simulink model "Boat_sim"  (Simulink 7.5)
settings: Solver=FixedStepDiscrete  StartTime=0.0  StopTime=1000  FixedStep=.01  RelTol=1e-3
InitFcn:
  | boat_constants
values from neighbouring files (symbols this model uses):
  C_d_sea_surge = 340    [boat_constants.m]
  d_prop = .4572    (= 0.4572)    [boat_constants.m]
  figure8_waypoints = int32([ ... (first row only)    [boat_constants.m]
  InitialPoint = 0    [boat_constants.m]    (also in l2plus.m)
  IPStar = 0    [boat_constants.m]    (also in l2plus.m)
  ISA_g = 9.815    [boat_constants.m]
  K_t = 0.5    [boat_constants.m]
  mass = 550    [boat_constants.m]
  MaxDwnPthStar = 1    [boat_constants.m]    (also in l2plus.m)
  OC2max = 49999    [boat_constants.m]    (also in simulation_constants.m)
  phi_0 = 0    [boat_constants.m]    (also in simulation_constants.m)
  rho_w = 1.03e3    (= 1030)    [boat_constants.m]
  sampling_waypoints = int32([ ... (first row only)    [boat_constants.m]
  switchDistance = 4    [boat_constants.m]    (also in l2plus.m)
  T_step = 0.01    [boat_constants.m]    (also in common.m)
  tanIntercept = tan( 45*pi/180 )    [boat_constants.m]    (also in l2plus.m)
  test_waypoints = int32([ ... (first row only)    [boat_constants.m]
  TStar = single(4.5)    [boat_constants.m]    (also in l2plus.m = single(2))
  Turn2Track = 0    [boat_constants.m]    (also in l2plus.m)
  wheelbase = 3.27    [boat_constants.m]
undefined symbols (not defined in the file or in its folder): clock, DiscIntNeverNeededParam, Earth, serial, WGS84
libraries: simulink x25, uSimLib x4, instrumentlib x3, aerolibconvert2 x2, aerolibtransform2 x1, aerolibanimutils x1, simulink_need_slupdate x1
(part 2 of 3)

== system Boat_sim/Subsystem/Log state data to workspace ==
  L2 : Inport
  gPos : Inport  Port=2
  head : Inport  Port=3
  lPos : Inport  Port=4
  vel : Inport  Port=5
  Build HIL sentence : Subsystem
  Pack : Stateflow chart  TreatAsAtomicUnit=on
  To Workspace2 : ToWorkspace  VariableName=state  SampleTime=-1  SaveFormat=Array
  wires:
  Pack/1(y) -> Build HIL sentence/1(data)
  Build HIL sentence/1(sent) -> To Workspace2/1
  L2/1 -> Pack/1(L2)
  gPos/1 -> Pack/2(gPos)
  head/1 -> Pack/3(head)
  lPos/1 -> Pack/4(lPos)
  vel/1 -> Pack/5(vel)

== system Boat_sim/Subsystem/Map from to 655..347 to -.7854..+.7854 ==
  In1 : Inport
  Bias1 : Bias  Bias=-501
  Data Type Conversion : DataTypeConversion  OutDataTypeMode=single  OutDataType=fixdt(1, 16)  OutScaling=2^0  OutDataTypeStr=single
  Gain : Gain  Gain=1/196  ParameterDataType=fixdt(1, 16)  ParameterScaling=2^0  OutDataType=fixdt(1, 16)  OutScaling=2^0
  Out1 : Outport
  wires:
  In1/1 -> Data Type Conversion/1
  Gain/1 -> Out1/1
  Bias1/1 -> Gain/1
  Data Type Conversion/1 -> Bias1/1

== system Boat_sim/Plant/Actuator Dynamics/Enabled Subsystem ==
  note: Map from 0,1 to -.02,.02
  In1 : Inport  OutDataType=fixdt(1, 16)  OutScaling=2^0
  Enable : EnablePort
  Bias : Bias  Bias=-1
  Data Type Conversion3 : DataTypeConversion  OutDataTypeMode=single  OutDataType=sfix(16)  OutScaling=2^0  OutDataTypeStr=single
  Gain : Gain  Gain=2  ParameterDataType=fixdt(1, 16)  ParameterScaling=2^0  OutDataTypeMode=double  OutDataType=fixdt(1, 16)  OutScaling=2^0  OutDataTypeStr=double
  Gain1 : Gain  Gain=.05  ParameterDataType=fixdt(1, 16)  ParameterScaling=2^0  OutDataType=fixdt(1, 16)  OutScaling=2^0
  Out1 : Outport  OutDataType=fixdt(1, 16)  OutScaling=2^0
  wires:
  In1/1 -> Data Type Conversion3/1
  Gain/1 -> Bias/1
  Bias/1 -> Gain1/1
  Gain1/1 -> Out1/1
  Data Type Conversion3/1 -> Gain/1

== system Boat_sim/Plant/Actuator Dynamics/Enabled Subsystem1 ==
  note: Map from 0,1 to -.5,.5
  In1 : Inport  OutDataType=fixdt(1, 16)  OutScaling=2^0
  Bias : Bias  Bias=-1
  Data Type Conversion : DataTypeConversion  OutDataTypeMode=single  OutDataType=fixdt(1, 16)  OutScaling=2^0  OutDataTypeStr=single
  Gain : Gain  Gain=2  ParameterDataType=fixdt(1, 16)  ParameterScaling=2^0  OutDataTypeMode=double  OutDataType=fixdt(1, 16)  OutScaling=2^0  OutDataTypeStr=double
  Shift Arithmetic : simulink/Logic and Bit Operations/Shift Arithmetic  SystemSampleTime=-1  nBitShiftRight=1  nBinPtShiftRight=0
  Out1 : Outport  OutDataType=fixdt(1, 16)  OutScaling=2^0
  wires:
  In1/1 -> Data Type Conversion/1
  Gain/1 -> Bias/1
  Bias/1 -> Shift Arithmetic/1
  Shift Arithmetic/1 -> Out1/1
  Data Type Conversion/1 -> Gain/1

== system Boat_sim/Plant/Actuator Dynamics/Second Order Linear Actuator1 ==
  Ac_dem : Inport  OutDataType=sfix(16)  OutScaling=2^0
  2*zeta * wn : Gain  Gain=2.0 * z_fin* wn_fin  ParameterDataType=sfix(16)  ParameterScaling=2^0  OutDataType=sfix(16)  OutScaling=2^0  SaturateOnIntegerOverflow=on  OutDataTypeStr=Inherit: Same as input  ParamDataTypeStr=Inherit: Same as input
  Discrete-Time Integrator1 : DiscreteIntegrator  SampleTime=-1  OutDataType=fixdt(1, 16)  OutScaling=2^0  UpperSaturationLimit=1  LowerSaturationLimit=-1  ICPrevOutput=DiscIntNeverNeededParam  ICPrevScaledInput=DiscIntNeverNeededParam
  Discrete-Time Integrator2 : DiscreteIntegrator  SampleTime=-1  OutDataType=fixdt(1, 16)  OutScaling=2^0  UpperSaturationLimit=1  LowerSaturationLimit=-1  ICPrevOutput=DiscIntNeverNeededParam  ICPrevScaledInput=DiscIntNeverNeededParam
  Sum2 : Sum  Inputs=|+-  OutDataType=sfix(16)  OutScaling=2^0  SaturateOnIntegerOverflow=on  InputSameDT=on  OutDataTypeStr=Inherit: Same as first input
  Sum3 : Sum  Inputs=|+-  OutDataType=sfix(16)  OutScaling=2^0  SaturateOnIntegerOverflow=on  InputSameDT=on  OutDataTypeStr=Inherit: Same as first input
  wn^2 : Gain  Gain=wn_fin* wn_fin  ParameterDataType=sfix(16)  ParameterScaling=2^0  OutDataType=sfix(16)  OutScaling=2^0  SaturateOnIntegerOverflow=on  OutDataTypeStr=Inherit: Same as input  ParamDataTypeStr=Inherit: Same as input
  Ac_ac : Outport  OutDataType=sfix(16)  OutScaling=2^0  InitialOutput=0
  wires:
  Discrete-Time Integrator1/1 -> Ac_ac/1, Sum3/2
  wn^2/1 -> Sum2/1
  Sum2/1 -> Discrete-Time Integrator2/1
  Discrete-Time Integrator2/1 -> 2*zeta * wn/1, Discrete-Time Integrator1/1
  2*zeta * wn/1 -> Sum2/2
  Ac_dem/1 -> Sum3/1
  Sum3/1 -> wn^2/1

== system Boat_sim/Plant/Actuator Dynamics/Second Order Linear Actuator2 ==
  Ac_dem : Inport  OutDataType=sfix(16)  OutScaling=2^0
  2*zeta * wn : Gain  Gain=2.0 * z_fin* wn_fin  ParameterDataType=sfix(16)  ParameterScaling=2^0  OutDataType=sfix(16)  OutScaling=2^0  SaturateOnIntegerOverflow=on  OutDataTypeStr=Inherit: Same as input  ParamDataTypeStr=Inherit: Same as input
  Discrete-Time Integrator1 : DiscreteIntegrator  SampleTime=-1  OutDataType=fixdt(1, 16)  OutScaling=2^0  UpperSaturationLimit=1  LowerSaturationLimit=-1  ICPrevOutput=DiscIntNeverNeededParam  ICPrevScaledInput=DiscIntNeverNeededParam
  Discrete-Time Integrator2 : DiscreteIntegrator  SampleTime=-1  OutDataType=fixdt(1, 16)  OutScaling=2^0  UpperSaturationLimit=1  LowerSaturationLimit=-1  ICPrevOutput=DiscIntNeverNeededParam  ICPrevScaledInput=DiscIntNeverNeededParam
  Sum2 : Sum  Inputs=|+-  OutDataType=sfix(16)  OutScaling=2^0  SaturateOnIntegerOverflow=on  InputSameDT=on  OutDataTypeStr=Inherit: Same as first input
  Sum3 : Sum  Inputs=|+-  OutDataType=sfix(16)  OutScaling=2^0  SaturateOnIntegerOverflow=on  InputSameDT=on  OutDataTypeStr=Inherit: Same as first input
  wn^2 : Gain  Gain=wn_fin* wn_fin  ParameterDataType=sfix(16)  ParameterScaling=2^0  OutDataType=sfix(16)  OutScaling=2^0  SaturateOnIntegerOverflow=on  OutDataTypeStr=Inherit: Same as input  ParamDataTypeStr=Inherit: Same as input
  Ac_ac : Outport  OutDataType=sfix(16)  OutScaling=2^0  InitialOutput=0
  wires:
  Discrete-Time Integrator1/1 -> Ac_ac/1, Sum3/2
  wn^2/1 -> Sum2/1
  Sum2/1 -> Discrete-Time Integrator2/1
  Discrete-Time Integrator2/1 -> 2*zeta * wn/1, Discrete-Time Integrator1/1
  2*zeta * wn/1 -> Sum2/2
  Ac_dem/1 -> Sum3/1
  Sum3/1 -> wn^2/1

== system Boat_sim/Plant/Actuator Dynamics/Second Order Linear Actuator3 ==
  Ac_dem : Inport  OutDataType=sfix(16)  OutScaling=2^0
  2*zeta * wn : Gain  Gain=2.0 * z_fin* wn_fin  ParameterDataType=sfix(16)  ParameterScaling=2^0  OutDataType=sfix(16)  OutScaling=2^0  SaturateOnIntegerOverflow=on  OutDataTypeStr=Inherit: Same as input  ParamDataTypeStr=Inherit: Same as input
  Discrete-Time Integrator1 : DiscreteIntegrator  SampleTime=-1  OutDataType=fixdt(1, 16)  OutScaling=2^0  UpperSaturationLimit=1  LowerSaturationLimit=-1  ICPrevOutput=DiscIntNeverNeededParam  ICPrevScaledInput=DiscIntNeverNeededParam
  Discrete-Time Integrator2 : DiscreteIntegrator  SampleTime=-1  OutDataType=fixdt(1, 16)  OutScaling=2^0  UpperSaturationLimit=1  LowerSaturationLimit=-1  ICPrevOutput=DiscIntNeverNeededParam  ICPrevScaledInput=DiscIntNeverNeededParam
  Sum2 : Sum  Inputs=|+-  OutDataType=sfix(16)  OutScaling=2^0  SaturateOnIntegerOverflow=on  InputSameDT=on  OutDataTypeStr=Inherit: Same as first input
  Sum3 : Sum  Inputs=|+-  OutDataType=sfix(16)  OutScaling=2^0  SaturateOnIntegerOverflow=on  InputSameDT=on  OutDataTypeStr=Inherit: Same as first input
  wn^2 : Gain  Gain=wn_fin* wn_fin  ParameterDataType=sfix(16)  ParameterScaling=2^0  OutDataType=sfix(16)  OutScaling=2^0  SaturateOnIntegerOverflow=on  OutDataTypeStr=Inherit: Same as input  ParamDataTypeStr=Inherit: Same as input
  Ac_ac : Outport  OutDataType=sfix(16)  OutScaling=2^0  InitialOutput=0
  wires:
  Discrete-Time Integrator1/1 -> Ac_ac/1, Sum3/2
  wn^2/1 -> Sum2/1
  Sum2/1 -> Discrete-Time Integrator2/1
  Discrete-Time Integrator2/1 -> 2*zeta * wn/1, Discrete-Time Integrator1/1
  2*zeta * wn/1 -> Sum2/2
  Ac_dem/1 -> Sum3/1
  Sum3/1 -> wn^2/1

== system Boat_sim/Plant/Actuator Dynamics/Subsystem ==
  note: This block stores the throttle speed. As the speed is only set intermittently,
      | the speed is saved to memory and constrantly output. It is only updated when
      | a properly packaged CAN message is delivered based on its ID and the trigger
      | bit.
  In1 : Inport
  Bus Selector2 : BusSelector  OutputSignals=identifier,trigger,data
  Data Store Memory : DataStoreMemory  DataStoreName=throttle_speed  WriteAfterWriteMsg=warning  WriteAfterReadMsg=warning  DataType=double  OutDataType=fixdt(1, 16)  OutScaling=2^0  OutDataTypeStr=double
  Data Store Read : DataStoreRead  Priority=2  DataStoreName=throttle_speed  SampleTime=T_step
  Data Type Conversion : DataTypeConversion  OutDataTypeMode=uint32  OutDataType=fixdt(1, 16)  OutScaling=2^0  OutDataTypeStr=uint32  RndMeth=Simplest
  If : If  NumInputs=2  IfExpression=u1 == hex2dec('301')  ShowElse=off
  If Action Subsystem : Subsystem  Priority=1  TreatAsAtomicUnit=on
  Scope1 : Scope
      settings: YMin=971.85  YMax=1074.15  SaveName=ScopeData2
  To Workspace : ToWorkspace  VariableName=t_data  SampleTime=-1  SaveFormat=Structure
  Out1 : Outport
  wires:
  In1/1 -> Bus Selector2/1
  Data Store Read/1 -> Out1/1, Scope1/1
  Bus Selector2/1 -> If/1  "<identifier>"
  Bus Selector2/2 -> Data Type Conversion/1  "<trigger>"
  If/1 -> If Action Subsystem/Action
  Bus Selector2/3 -> If Action Subsystem/1(In1), To Workspace/1  "<data>"
  Data Type Conversion/1 -> If/2

== system Boat_sim/Plant/Actuator Dynamics/Subsystem1 ==
  note: This block simulates the stepper motor driver board logic for stepping the motor.
      | The enable line must be low, it's active low, and a pulse train must be received. As
      | the enable line is always low to provide holding torque, the lines specifying a pulse
      | train must are therefore checked to confirm that the rudder should be moving. The
      | exact values of both the up and period signals are unimportant, so they're just
      | compared to zero.
  e : Inport
  u : Inport  Port=2
  p : Inport  Port=3
  Compare To Zero : simulink/Logic and Bit Operations/Compare To Zero  SystemSampleTime=-1  relop=~=  LogicOutDataTypeMode=boolean
  Compare To Zero1 : simulink/Logic and Bit Operations/Compare To Zero  SystemSampleTime=-1  relop=~=  LogicOutDataTypeMode=boolean
  Logical Operator : Logic  Operator=NOT  AllPortsSameDT=off  OutDataTypeMode=boolean  LogicDataType=fixdt(0, 8)  OutDataTypeStr=boolean
  Logical Operator1 : Logic  Inputs=3  AllPortsSameDT=off  OutDataTypeMode=boolean  LogicDataType=fixdt(0, 8)  OutDataTypeStr=boolean
  Out1 : Outport
  wires:
  e/1 -> Logical Operator/1
  Logical Operator1/1 -> Out1/1
  p/1 -> Compare To Zero/1
  Compare To Zero/1 -> Logical Operator1/3
  Compare To Zero1/1 -> Logical Operator1/2
  u/1 -> Compare To Zero1/1
  Logical Operator/1 -> Logical Operator1/1

== system Boat_sim/Plant/Generate sensor data from actuator position/Map from +-.7854 to 655..347 ==
  In1 : Inport
  Bias1 : Bias  Bias=501
  Data Type Conversion : DataTypeConversion  OutDataTypeMode=uint16  OutDataType=fixdt(1, 16)  OutScaling=2^0  OutDataTypeStr=uint16
  Gain1 : Gain  Gain=196  ParameterDataType=fixdt(1, 16)  ParameterScaling=2^0  OutDataType=fixdt(1, 16)  OutScaling=2^0
  Out1 : Outport
  wires:
  Bias1/1 -> Data Type Conversion/1
  In1/1 -> Gain1/1
  Data Type Conversion/1 -> Out1/1
  Gain1/1 -> Bias1/1

== system Boat_sim/Plant/Generate sensor data from actuator position/Map from -1..1 to -1023..1023 ==
  In1 : Inport
  Data Type Conversion : DataTypeConversion  OutDataTypeMode=int16  OutDataType=fixdt(1, 16)  OutScaling=2^0  OutDataTypeStr=int16  RndMeth=Simplest
  Gain : Gain  Gain=1023  ParameterDataType=fixdt(1, 16)  ParameterScaling=2^0  OutDataType=fixdt(1, 16)  OutScaling=2^0
  Out1 : Outport
  wires:
  Gain/1 -> Data Type Conversion/1
  In1/1 -> Gain/1
  Data Type Conversion/1 -> Out1/1

== system Boat_sim/Plant/Generate sensor data from actuator position/Map from -1..1 to 620..313 ==
  In1 : Inport
  Bias : Bias  Bias=466.5
  Data Type Conversion : DataTypeConversion  OutDataTypeMode=uint16  OutDataType=fixdt(1, 16)  OutScaling=2^0  OutDataTypeStr=uint16
  Gain : Gain  Gain=-153.5  ParameterDataType=fixdt(1, 16)  ParameterScaling=2^0  OutDataType=fixdt(1, 16)  OutScaling=2^0
  Out1 : Outport
  wires:
  Data Type Conversion/1 -> Out1/1
  In1/1 -> Gain/1
  Bias/1 -> Data Type Conversion/1
  Gain/1 -> Bias/1

== system Boat_sim/Subsystem/Autonomous Controller/Ballast Command ==
  Bus Creator : BusCreator  Inputs=2
  Constant : Constant  Value=0  OutDataTypeMode=boolean  OutDataType=fixdt(1, 16)  OutScaling=2^0  OutDataTypeStr=boolean
  Constant1 : Constant  Value=0  OutDataTypeMode=boolean  OutDataType=fixdt(1, 16)  OutScaling=2^0  OutDataTypeStr=boolean
  c_ballast : Outport
  wires:
  Constant1/1 -> Bus Creator/2  "direction"
  Constant/1 -> Bus Creator/1  "enable"
  Bus Creator/1 -> c_ballast/1

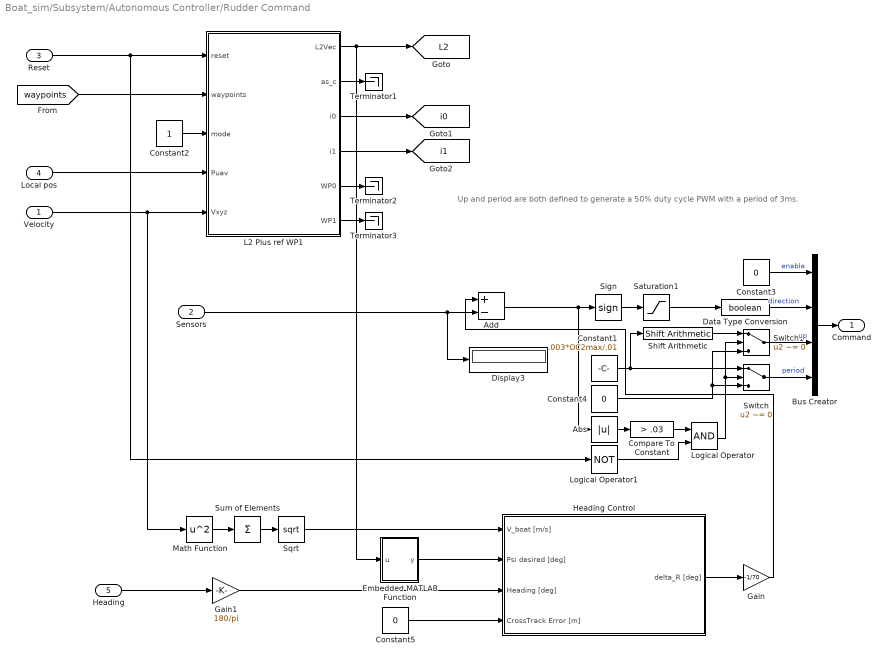
== system Boat_sim/Subsystem/Autonomous Controller/Rudder Command ==
  note: Up and period are both defined to generate a 50% duty cycle PWM with
      | a period of 3ms.
  Velocity : Inport
  Sensors : Inport  Port=2
  Reset : Inport  Port=3
  Local pos : Inport  Port=4
  Heading : Inport  Port=5
  Abs : Abs  OutDataType=fixdt(1, 16)  OutScaling=2^0
  Add : Sum  Inputs=+-  OutDataType=fixdt(1, 16)  OutScaling=2^-10
  Bus Creator : BusCreator
  Compare To Constant : simulink/Logic and Bit Operations/Compare To Constant  SystemSampleTime=-1  relop=>  const=.03  LogicOutDataTypeMode=boolean
  Constant1 : Constant  Value=.003*OC2max/.01  OutDataTypeMode=uint16  OutDataType=sfix(16)  OutScaling=2^0  OutDataTypeStr=uint16
  Constant2 : Constant  OutDataTypeMode=uint8  OutDataType=sfix(16)  OutScaling=2^0  OutDataTypeStr=uint8
  Constant3 : Constant  Value=0  OutDataTypeMode=boolean  OutDataType=sfix(16)  OutScaling=2^0  OutDataTypeStr=boolean
  Constant4 : Constant  Value=0  OutDataTypeMode=uint16  OutDataType=sfix(16)  OutScaling=2^0  OutDataTypeStr=uint16
  Constant5 : Constant  Value=0  OutDataTypeMode=uint8  OutDataType=sfix(16)  OutScaling=2^0  OutDataTypeStr=uint8
  Data Type Conversion : DataTypeConversion  OutDataTypeMode=boolean  OutDataType=fixdt(1, 16)  OutScaling=2^0  OutDataTypeStr=boolean  RndMeth=Simplest
  Display3 : Display
  Embedded MATLAB Function : Stateflow chart  TreatAsAtomicUnit=on
  Gain : Gain  Gain=-1/70  ParameterDataType=fixdt(1, 16)  ParameterScaling=2^0  OutDataType=fixdt(1, 16)  OutScaling=2^0
  Gain1 : Gain  Gain=180/pi  ParameterDataType=fixdt(1, 16)  ParameterScaling=2^0  OutDataType=fixdt(1, 16)  OutScaling=2^0
  Heading Control : Subsystem
  L2 Plus ref WP1 : Stateflow chart  TreatAsAtomicUnit=on
  Logical Operator : Logic  AllPortsSameDT=off  OutDataTypeMode=boolean  LogicDataType=fixdt(0, 8)  OutDataTypeStr=boolean
  Logical Operator1 : Logic  Operator=NOT  Inputs=1  AllPortsSameDT=off  OutDataTypeMode=boolean  LogicDataType=fixdt(0, 8)  OutDataTypeStr=boolean
  Math Function : Math  Operator=square  OutDataType=fixdt(1, 16)  OutScaling=2^0  SaturateOnIntegerOverflow=on
  Saturation1 : Saturate  UpperLimit=1  LowerLimit=0  OutDataTypeStr=Inherit: Inherit via back propagation
  Shift Arithmetic : simulink/Logic and Bit Operations/Shift Arithmetic  SystemSampleTime=-1  nBitShiftRight=1  nBinPtShiftRight=0
  Sign : Signum
  Sqrt : Sqrt  SaturateOnIntegerOverflow=on
  Sum of Elements : Sum  Inputs=+  OutDataType=fixdt(1, 16)  OutScaling=2^-10
  Switch : Switch  Criteria=u2 ~= 0  OutDataType=fixdt(1, 16)  OutScaling=2^0
  Switch1 : Switch  Criteria=u2 ~= 0  OutDataType=fixdt(1, 16)  OutScaling=2^0
  Terminator1 : Terminator
  Terminator2 : Terminator
  Terminator3 : Terminator
  Command : Outport
  tag scope: L2=global, i0=global, i1=global
  wires:
  Add/1 -> Abs/1, Sign/1
  Embedded MATLAB Function/1(y) -> Heading Control/2(Psi desired [deg])
  Gain1/1 -> Heading Control/3(Heading [deg])
  Gain/1 -> Add/1
  Heading Control/1(delta_R [deg]) -> Gain/1
  Sum of Elements/1 -> Sqrt/1
  Math Function/1 -> Sum of Elements/1
  Sqrt/1 -> Heading Control/1(V_boat [m/s])
  Constant5/1 -> Heading Control/4(CrossTrack Error [m])
  Heading/1 -> Gain1/1
  [waypoints] -> L2 Plus ref WP1/2(waypoints)
  Logical Operator1/1 -> Logical Operator/2
  Logical Operator/1 -> Switch1/2, Switch/2
  Compare To Constant/1 -> Logical Operator/1
  L2 Plus ref WP1/4(i1) -> [i1]
  L2 Plus ref WP1/3(i0) -> [i0]
  Local pos/1 -> L2 Plus ref WP1/4(Puav)
  Reset/1 -> Logical Operator1/1, L2 Plus ref WP1/1(reset)
  Constant4/1 -> Switch1/3, Switch/3
  Switch1/1 -> Bus Creator/3  "up"
  Switch/1 -> Bus Creator/4  "period"
  Shift Arithmetic/1 -> Switch1/1
  Abs/1 -> Compare To Constant/1
  Constant1/1 -> Switch/1, Shift Arithmetic/1
  Constant3/1 -> Bus Creator/1  "enable"
  Velocity/1 -> Math Function/1, L2 Plus ref WP1/5(Vxyz)
  L2 Plus ref WP1/1(L2Vec) -> Embedded MATLAB Function/1(u), [L2]
  Constant2/1 -> L2 Plus ref WP1/3(mode)
  Sign/1 -> Saturation1/1
  Saturation1/1 -> Data Type Conversion/1
  Bus Creator/1 -> Command/1
  Sensors/1 -> Add/2, Display3/1
  Data Type Conversion/1 -> Bus Creator/2  "direction"
  L2 Plus ref WP1/2(as_c) -> Terminator1/1
  L2 Plus ref WP1/5(WP0) -> Terminator2/1
  L2 Plus ref WP1/6(WP1) -> Terminator3/1

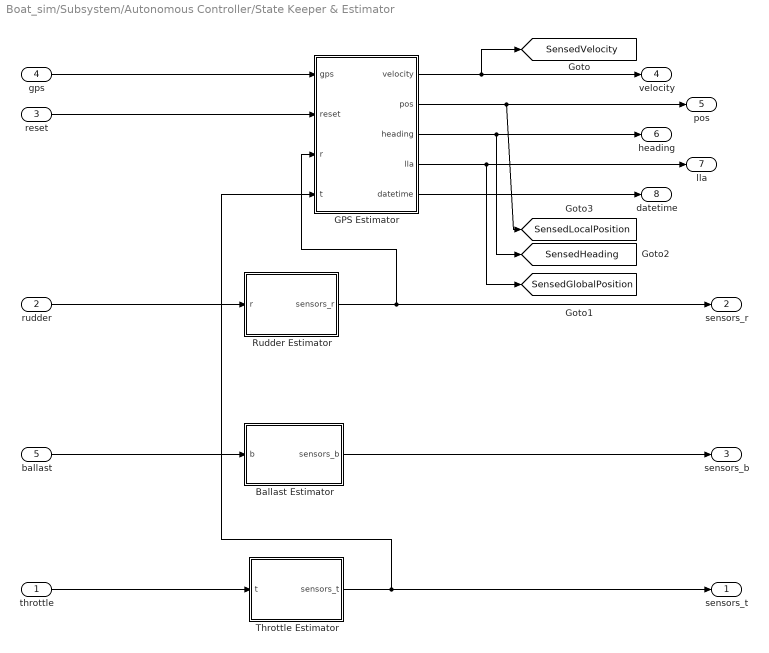
== system Boat_sim/Subsystem/Autonomous Controller/State Keeper & Estimator ==
  throttle : Inport
  rudder : Inport  Port=2
  reset : Inport  Port=3
  gps : Inport  Port=4
  ballast : Inport  Port=5
  Ballast Estimator : Subsystem
  GPS Estimator : Subsystem
  Rudder Estimator : Subsystem
  Throttle Estimator : Subsystem
  sensors_t : Outport
  sensors_r : Outport  Port=2
  sensors_b : Outport  Port=3
  velocity : Outport  Port=4
  pos : Outport  Port=5
  heading : Outport  Port=6
  lla : Outport  Port=7
  datetime : Outport  Port=8
  tag scope: SensedGlobalPosition=global, SensedHeading=global, SensedLocalPosition=global, SensedVelocity=global
  wires:
  Throttle Estimator/1(sensors_t) -> GPS Estimator/4(t), sensors_t/1
  Ballast Estimator/1(sensors_b) -> sensors_b/1
  Rudder Estimator/1(sensors_r) -> GPS Estimator/3(r), sensors_r/1
  GPS Estimator/5(datetime) -> datetime/1
  GPS Estimator/4(lla) -> lla/1, [SensedGlobalPosition]
  GPS Estimator/3(heading) -> [SensedHeading], heading/1
  GPS Estimator/2(pos) -> [SensedLocalPosition], pos/1
  gps/1 -> GPS Estimator/1(gps)
  GPS Estimator/1(velocity) -> [SensedVelocity], velocity/1
  reset/1 -> GPS Estimator/2(reset)
  throttle/1 -> Throttle Estimator/1(t)
  ballast/1 -> Ballast Estimator/1(b)
  rudder/1 -> Rudder Estimator/1(r)

== system Boat_sim/Subsystem/Autonomous Controller/Throttle Command ==
  sensors : Inport
  reset : Inport  Port=2
  Bus Creator : BusCreator
  Constant1 : Constant  Value=0  OutDataTypeMode=int16  OutDataType=sfix(16)  OutScaling=2^0  OutDataTypeStr=int16
  Constant5 : Constant  Value=1000  OutDataTypeMode=int16  OutDataType=sfix(16)  OutScaling=2^0  OutDataTypeStr=int16
  Mux Everything : Subsystem
  Switch : Switch  Criteria=u2 > Threshold  OutDataType=fixdt(1, 16)  OutScaling=2^0
  Terminator : Terminator
  Trigger Events : Subsystem
  command : Outport  OutDataType=sfix(16)  OutScaling=2^0
  wires:
  Constant5/1 -> Switch/3
  Constant1/1 -> Switch/1
  Switch/1 -> Trigger Events/1(RC Throttle), Mux Everything/4(Throttle)
  Mux Everything/4(trig) -> Bus Creator/4  "trigger"
  Mux Everything/3(size) -> Bus Creator/3  "size"
  Mux Everything/2(data) -> Bus Creator/2  "data"
  Mux Everything/1(iden) -> Bus Creator/1  "identifier"
  reset/1 -> Switch/2, Trigger Events/2(Reset)
  Trigger Events/2(Disable) -> Mux Everything/2(disable)
  Trigger Events/3(Enable) -> Mux Everything/3(enable)
  Trigger Events/1(Change Speed) -> Mux Everything/1(speed)
  Bus Creator/1 -> command/1
  sensors/1 -> Terminator/1

== system Boat_sim/Subsystem/Log state data to workspace/Build HIL sentence ==
  data : Inport
  Bitwise Operator : simulink/Logic and Bit Operations/Bitwise Operator  logicop=XOR  UseBitMask=off  BitMask=bin2dec('11011001')  BitMaskRealWorld=Stored Integer
  Constant : Constant  Value=37  OutDataTypeMode=uint8  OutDataType=fixdt(1, 16)  OutScaling=2^0  OutDataTypeStr=uint8
  Constant1 : Constant  Value=38  OutDataTypeMode=uint8  OutDataType=fixdt(1, 16)  OutScaling=2^0  OutDataTypeStr=uint8
  Constant2 : Constant  Value=94  OutDataTypeMode=uint8  OutDataType=fixdt(1, 16)  OutScaling=2^0  OutDataTypeStr=uint8
  Constant3 : Constant  Value=38  OutDataTypeMode=uint8  OutDataType=fixdt(1, 16)  OutScaling=2^0  OutDataTypeStr=uint8
  Constant4 : Constant  Value=3  OutDataTypeMode=uint8  OutDataType=fixdt(1, 16)  OutScaling=2^0  OutDataTypeStr=uint8
  Mux2 : Mux  Inputs=2
  Pack : Stateflow chart  TreatAsAtomicUnit=on
  sent : Outport
  wires:
  data/1 -> Mux2/2, Pack/4(d)
  Constant/1 -> Pack/1(a)
  Constant1/1 -> Pack/2(b)
  Pack/1(y) -> sent/1
  Constant4/1 -> Mux2/1, Pack/3(c)
  Constant2/1 -> Pack/5(e)
  Constant3/1 -> Pack/6(f)
  Bitwise Operator/1 -> Pack/7(g)
  Mux2/1 -> Bitwise Operator/1

== system Boat_sim/Plant/Actuator Dynamics/Subsystem/If Action Subsystem ==
  In1 : Inport  OutDataType=fixdt(1, 16)  OutScaling=2^0
  Action Port : ActionPort  ActionType=then
  Bitwise Operator : simulink/Logic and Bit Operations/Bitwise Operator  logicop=OR  UseBitMask=off  NumInputPorts=2  BitMask=bin2dec('11011001')  BitMaskRealWorld=Stored Integer
  Data Store Write : DataStoreWrite  DataStoreName=throttle_speed  SampleTime=-1
  Data Type Conversion : DataTypeConversion  OutDataTypeMode=uint16  OutDataType=fixdt(1, 16)  OutScaling=2^0  OutDataTypeStr=uint16  ConvertRealWorld=Stored Integer (SI)
  Data Type Conversion2 : DataTypeConversion  OutDataTypeMode=double  OutDataType=sfix(16)  OutScaling=2^0  OutDataTypeStr=double  LockScale=on
  Demux : Demux  Outputs=2
  Gain : Gain  Gain=1/1023  ParameterDataType=fixdt(1, 16)  ParameterScaling=2^0  OutDataType=fixdt(1, 16)  OutScaling=2^0
  Selector2 : Selector  InputPortWidth=6  IndexOptions=Index vector (dialog)  Indices=[4 3]  OutputSizes=1
  Shift Arithmetic : simulink/Logic and Bit Operations/Shift Arithmetic  SystemSampleTime=-1  nBitShiftRight=-8  nBinPtShiftRight=0
  wires:
  In1/1 -> Selector2/1
  Data Type Conversion2/1 -> Gain/1
  Gain/1 -> Data Store Write/1
  Selector2/1 -> Data Type Conversion/1
  Bitwise Operator/1 -> Data Type Conversion2/1
  Data Type Conversion/1 -> Demux/1
  Demux/1 -> Bitwise Operator/1
  Demux/2 -> Shift Arithmetic/1
  Shift Arithmetic/1 -> Bitwise Operator/2

== system Boat_sim/Subsystem/Autonomous Controller/Rudder Command/Heading Control ==
  note: Heading Error
  V_boat [m/s] : Inport  OutDataType=sfix(16)  OutScaling=2^0
  Psi desired [deg] : Inport  Port=2  OutDataType=sfix(16)  OutScaling=2^0
  Heading [deg] : Inport  Port=3  OutDataType=sfix(16)  OutScaling=2^0
  CrossTrack Error [m] : Inport  Port=4  OutDataType=sfix(16)  OutScaling=2^0
  Abs : Abs
  Angle Conversion : aerolibconvert2/Angle Conversion  SystemSampleTime=-1  IU=deg  OU=rad
  Angle Conversion1 : aerolibconvert2/Angle Conversion  SystemSampleTime=-1  IU=rad  OU=deg
  Constant : Constant  OutDataType=sfix(16)  OutScaling=2^0
  Divide : Product  Inputs=*/  OutDataType=sfix(16)  OutScaling=2^-10
  Fcn2 : Fcn  Expr=(u<-180)*360 + u + (u>180)*(-360)
  Kpsi : Gain  ParameterDataType=sfix(16)  ParameterScaling=2^0  OutDataType=sfix(16)  OutScaling=2^0
  MinMax : MinMax  Function=max  Inputs=2  OutDataType=sfix(16)  OutScaling=2^0
  Product : Product  OutDataType=sfix(16)  OutScaling=2^0  RndMeth=Zero
  Saturation : Saturate  UpperLimit=70  LowerLimit=-70
  Sign : Signum
  Sum : Sum  Inputs=-+|  OutDataType=sfix(16)  OutScaling=2^0
  Terminator : Terminator
  delta_R [deg] : Outport  OutDataType=sfix(16)  OutScaling=2^0
  wires:
  Fcn2/1 -> Angle Conversion/1
  Angle Conversion/1 -> Kpsi/1
  V_boat [m/s]/1 -> Abs/1, Sign/1
  Product/1 -> Angle Conversion1/1
  Kpsi/1 -> Product/2
  Sign/1 -> Product/1
  Angle Conversion1/1 -> Divide/1
  Divide/1 -> Saturation/1
  Abs/1 -> MinMax/1
  Constant/1 -> MinMax/2
  Saturation/1 -> delta_R [deg]/1
  MinMax/1 -> Divide/2
  CrossTrack Error [m]/1 -> Terminator/1
  Psi desired [deg]/1 -> Sum/1
  Heading [deg]/1 -> Sum/2
  Sum/1 -> Fcn2/1

== system Boat_sim/Subsystem/Autonomous Controller/State Keeper & Estimator/Ballast Estimator ==
  b : Inport
  Bus Selector1 : BusSelector  OutputSignals=position
  sensors_b : Outport
  wires:
  Bus Selector1/1 -> sensors_b/1  "<position>"
  b/1 -> Bus Selector1/1

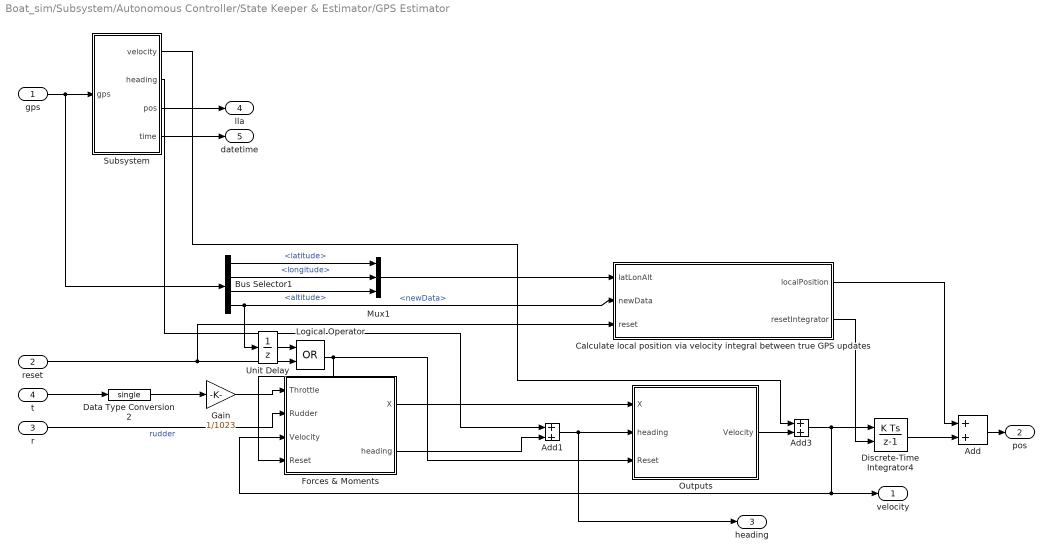
== system Boat_sim/Subsystem/Autonomous Controller/State Keeper & Estimator/GPS Estimator ==
  gps : Inport
  reset : Inport  Port=2  OutDataType=fixdt(1, 16)  OutScaling=2^0
  r : Inport  Port=3  OutDataType=fixdt(1, 16)  OutScaling=2^0
  t : Inport  Port=4  OutDataType=fixdt(1, 16)  OutScaling=2^0
  Add : Sum  OutDataType=fixdt(1, 16)  OutScaling=2^-10
  Add1 : Sum  OutDataType=fixdt(1, 16)  OutScaling=2^-10
  Add3 : Sum  OutDataType=fixdt(1, 16)  OutScaling=2^-10
  Bus Selector1 : BusSelector  OutputSignals=latitude,longitude,altitude,newData
  Calculate local position via velocity integral between true GPS updates : Stateflow chart  TreatAsAtomicUnit=on
  Data Type Conversion2 : DataTypeConversion  OutDataTypeMode=single  OutDataType=sfix(16)  OutScaling=2^0  OutDataTypeStr=single  LockScale=on
  Discrete-Time Integrator4 : DiscreteIntegrator  ExternalReset=level  SampleTime=-1  OutDataType=fixdt(1, 16)  OutScaling=2^0  ICPrevOutput=DiscIntNeverNeededParam  ICPrevScaledInput=DiscIntNeverNeededParam
  Forces & Moments : Subsystem
  Gain : Gain  Gain=1/1023  ParameterDataType=fixdt(1, 16)  ParameterScaling=2^0  OutDataType=fixdt(1, 16)  OutScaling=2^0
  Logical Operator : Logic  Operator=OR  AllPortsSameDT=off  OutDataTypeMode=boolean  LogicDataType=fixdt(0, 8)  OutDataTypeStr=boolean
  Mux1 : Mux  Inputs=3
  Outputs : Subsystem
  Subsystem : Subsystem
  Unit Delay : UnitDelay  SampleTime=-1
  velocity : Outport
  pos : Outport  Port=2
  heading : Outport  Port=3
  lla : Outport  Port=4
  datetime : Outport  Port=5
  wires:
  Unit Delay/1 -> Logical Operator/1
  Add3/1 -> Forces & Moments/3(Velocity), velocity/1, Discrete-Time Integrator4/1
  Outputs/1(Velocity) -> Add3/2
  Logical Operator/1 -> Forces & Moments/4(Reset), Outputs/3(Reset)
  Calculate local position via velocity integral between true GPS updates/1(localPosition) -> Add/1
  Calculate local position via velocity integral between true GPS updates/2(resetIntegrator) -> Discrete-Time Integrator4/2
  Mux1/1 -> Calculate local position via velocity integral between true GPS updates/1(latLonAlt)
  Bus Selector1/4 -> Unit Delay/1, Calculate local position via velocity integral between true GPS updates/2(newData)  "<newData>"
  Bus Selector1/3 -> Mux1/3  "<altitude>"
  Bus Selector1/2 -> Mux1/2  "<longitude>"
  Bus Selector1/1 -> Mux1/1  "<latitude>"
  Add/1 -> pos/1
  Discrete-Time Integrator4/1 -> Add/2
  t/1 -> Data Type Conversion2/1
  Gain/1 -> Forces & Moments/1(Throttle)
  Data Type Conversion2/1 -> Gain/1
  Forces & Moments/2(heading) -> Add1/2
  Add1/1 -> heading/1, Outputs/2(heading)
  reset/1 -> Calculate local position via velocity integral between true GPS updates/3(reset), Logical Operator/2
  r/1 -> Forces & Moments/2(Rudder)  "rudder"
  Forces & Moments/1(X) -> Outputs/1(X)
  Subsystem/4(time) -> datetime/1
  Subsystem/3(pos) -> lla/1
  Subsystem/2(heading) -> Add1/1
  Subsystem/1(velocity) -> Add3/1
  gps/1 -> Bus Selector1/1, Subsystem/1(gps)

== system Boat_sim/Subsystem/Autonomous Controller/State Keeper & Estimator/Rudder Estimator ==
  r : Inport
  sensors_r : Outport
  wires:
  r/1 -> sensors_r/1

== system Boat_sim/Subsystem/Autonomous Controller/State Keeper & Estimator/Throttle Estimator ==
  t : Inport
  sensors_t : Outport
  wires:
  t/1 -> sensors_t/1

== system Boat_sim/Subsystem/Autonomous Controller/Throttle Command/Mux Everything ==
  speed : Inport  OutDataType=sfix(16)  OutScaling=2^0
  disable : Inport  Port=2  OutDataType=sfix(16)  OutScaling=2^0
  enable : Inport  Port=3  OutDataType=sfix(16)  OutScaling=2^0
  Throttle : Inport  Port=4  OutDataType=sfix(16)  OutScaling=2^0
  0x300 : Constant  Value=768  OutDataTypeMode=uint32  OutDataType=sfix(16)  OutScaling=2^0  OutDataTypeStr=uint32
  0x301 : Constant  Value=769  OutDataTypeMode=uint32  OutDataType=sfix(16)  OutScaling=2^0  OutDataTypeStr=uint32
  Build speed command : Subsystem
  Disable motor : Constant  Value=[0 0 0 0 64 0]  OutDataTypeMode=uint8  OutDataType=sfix(16)  OutScaling=2^0  OutDataTypeStr=uint8
  Enable motor : Constant  Value=[0 0 0 0 32 0]  OutDataTypeMode=uint8  OutDataType=sfix(16)  OutScaling=2^0  OutDataTypeStr=uint8
  Logical Operator1 : Logic  Operator=OR  AllPortsSameDT=off  OutDataTypeMode=boolean  OutDataTypeStr=boolean
  Message Length1 : Probe  ProbeSampleTime=off  ProbeComplexSignal=off  ProbeWidthDataType=uint8
  Multiport Switch : MultiPortSwitch  zeroidx=off
  Multiport Switch1 : MultiPortSwitch  zeroidx=off
  Select data packet : Stateflow chart  TreatAsAtomicUnit=on
  Switch : Switch  Criteria=u2 ~= 0
  To Workspace1 : ToWorkspace  VariableName=trig  SampleTime=-1  SaveFormat=Array
  To Workspace3 : ToWorkspace  VariableName=sel  SampleTime=-1  SaveFormat=Array
  iden : Outport  OutDataType=sfix(16)  OutScaling=2^0
  data : Outport  Port=2  OutDataType=sfix(16)  OutScaling=2^0
  size : Outport  Port=3  OutDataType=sfix(16)  OutScaling=2^0
  trig : Outport  Port=4  OutDataType=sfix(16)  OutScaling=2^0
  wires:
  Build speed command/1(msg) -> Multiport Switch/4
  speed/1 -> Multiport Switch1/4
  Multiport Switch1/1 -> To Workspace1/1, trig/1
  Select data packet/1(y) -> To Workspace3/1, Multiport Switch1/1, Multiport Switch/1
  Logical Operator1/1 -> Switch/2
  enable/1 -> Multiport Switch1/3, Select data packet/2(en), Logical Operator1/2
  disable/1 -> Multiport Switch1/2, Select data packet/1(dis), Logical Operator1/1
  Switch/1 -> iden/1
  0x301/1 -> Switch/3
  0x300/1 -> Switch/1
  Message Length1/1 -> size/1
  Multiport Switch/1 -> data/1, Message Length1/1
  Throttle/1 -> Build speed command/1(CC)
  Disable motor/1 -> Multiport Switch/2
  Enable motor/1 -> Multiport Switch/3

== system Boat_sim/Subsystem/Autonomous Controller/Throttle Command/Trigger Events ==
  RC Throttle : Inport  OutDataType=sfix(16)  OutScaling=2^0
  Reset : Inport  Port=2  OutDataType=sfix(16)  OutScaling=2^0
  Data Type Conversion1 : DataTypeConversion  OutDataTypeMode=boolean  OutDataType=sfix(16)  OutScaling=2^0  OutDataTypeStr=boolean
  Data Type Conversion2 : DataTypeConversion  OutDataTypeMode=boolean  OutDataType=sfix(16)  OutScaling=2^0  OutDataTypeStr=boolean
  Data Type Conversion3 : DataTypeConversion  OutDataTypeMode=boolean  OutDataType=sfix(16)  OutScaling=2^0  OutDataTypeStr=boolean
  Detect Change : simulink/Logic and Bit Operations/Detect Change  SystemSampleTime=-1  vinit=0
  Detect Fall Nonpositive : simulink/Logic and Bit Operations/Detect Fall Nonpositive  SystemSampleTime=-1  vinit=0
  Detect Rise Positive : simulink/Logic and Bit Operations/Detect Rise Positive  SystemSampleTime=-1  vinit=0
  Shift Arithmetic : simulink/Logic and Bit Operations/Shift Arithmetic  SystemSampleTime=-1  nBitShiftRight=2  nBinPtShiftRight=0
  Weighted Moving Average : simulink_need_slupdate/Weighted Moving Average  mgainval=[.5 .5]  vinit=0.0  samptime=-1  OutDataTypeStr=Inherit: Inherit via back propagation  OutDataType=sfix(16)  OutScaling=2^-10  DoSatur=off  GainDataType=uint(16)  MatRadixGroup=Best Precision: Matrix-wise  GainScaling=2^-10
  Change Speed : Outport  OutDataType=sfix(16)  OutScaling=2^0
  Disable : Outport  Port=2  OutDataType=sfix(16)  OutScaling=2^0
  Enable : Outport  Port=3  OutDataType=sfix(16)  OutScaling=2^0
  wires:
  Data Type Conversion1/1 -> Disable/1
  Data Type Conversion2/1 -> Enable/1
  Data Type Conversion3/1 -> Change Speed/1
  Detect Rise Positive/1 -> Data Type Conversion1/1
  Detect Fall Nonpositive/1 -> Data Type Conversion2/1
  Reset/1 -> Detect Rise Positive/1, Detect Fall Nonpositive/1
  Shift Arithmetic/1 -> Weighted Moving Average/1
  Weighted Moving Average/1 -> Detect Change/1
  Detect Change/1 -> Data Type Conversion3/1
  RC Throttle/1 -> Shift Arithmetic/1

== system Boat_sim/Subsystem/Autonomous Controller/State Keeper & Estimator/GPS Estimator/Forces & Moments ==
  note: This subsystem computes the forward force, heading and roll of the boat that
      | is to be expected based on the current state. The model for these calculations
      | is based off of the calculations performed in the original WG1 boat model.
      |
      | The eventual goal of this subsystem to provide all 6 forces and moments for the
      | boat, instead of only one + final orientation parameters.
  Throttle : Inport  OutDataType=sfix(16)  OutScaling=2^0
  Rudder : Inport  Port=2  OutDataType=sfix(16)  OutScaling=2^0
  Velocity : Inport  Port=3  OutDataType=sfix(16)  OutScaling=2^0
  Reset : Inport  Port=4  OutDataType=sfix(16)  OutScaling=2^0
  C_d : Gain  Gain=C_d_sea_surge  ParameterDataType=sfix(16)  ParameterScaling=2^0  OutDataType=sfix(16)  OutScaling=2^0
  Convert to RPS : Gain  Gain=450/60  ParameterDataType=sfix(16)  ParameterScaling=2^0  OutDataType=sfix(16)  OutScaling=2^0
  Convert to force : Fcn  Expr=rho_w*(d_prop^4)*K_t*abs(u)*u
  Discrete-Time Integrator : DiscreteIntegrator  ExternalReset=level  SampleTime=-1  OutDataType=fixdt(1, 16)  OutScaling=2^0  ICPrevOutput=DiscIntNeverNeededParam  ICPrevScaledInput=DiscIntNeverNeededParam
  Divide by wheelbase : Gain  Gain=1/wheelbase  ParameterDataType=sfix(16)  ParameterScaling=2^0  OutDataType=sfix(16)  OutScaling=2^0
  Fcn : Fcn  Expr=sqrt(u(1)^2+u(2)^2+u(3)^2)
  Fcn3 : Fcn  Expr=abs(u)*u
  Initial heading : Constant  Value=phi_0  OutDataTypeMode=single  OutDataType=sfix(16)  OutScaling=2^0  OutDataTypeStr=single
  Product3 : Product  OutDataType=sfix(16)  OutScaling=2^0  RndMeth=Zero
  Sum1 : Sum  Inputs=|+-  OutDataType=sfix(16)  OutScaling=2^0
  Sum2 : Sum  OutDataType=sfix(16)  OutScaling=2^0
  Trigonometric Function2 : Trigonometry  Operator=tan  OutputSignalType=real
  X : Outport  OutDataType=sfix(16)  OutScaling=2^0
  heading : Outport  Port=2  OutDataType=sfix(16)  OutScaling=2^0
  wires:
  Reset/1 -> Discrete-Time Integrator/2
  Convert to RPS/1 -> Convert to force/1  "RPS"
  Fcn3/1 -> C_d/1
  C_d/1 -> Sum1/2
  Convert to force/1 -> Sum1/1
  Velocity/1 -> Fcn/1
  Throttle/1 -> Convert to RPS/1
  Sum1/1 -> X/1
  Fcn/1 -> Fcn3/1, Product3/1
  Rudder/1 -> Trigonometric Function2/1
  Trigonometric Function2/1 -> Product3/2
  Product3/1 -> Divide by wheelbase/1
  Divide by wheelbase/1 -> Discrete-Time Integrator/1
  Discrete-Time Integrator/1 -> Sum2/1
  Initial heading/1 -> Sum2/2
  Sum2/1 -> heading/1

== system Boat_sim/Subsystem/Autonomous Controller/State Keeper & Estimator/GPS Estimator/Outputs ==
  note: This subsystem converts the heading and forward forces into a current position
      |  defined by the latitude and longitude. It does this by using the current LLA
      | as a reference for a flat plane. The local displacement during the last timestep
      | is mapped into ECEF coordinates and then to LLA from there to provide the new
      | location. Output is in degrees.
  X : Inport  OutDataType=sfix(16)  OutScaling=2^0
  heading : Inport  Port=2  OutDataType=sfix(16)  OutScaling=2^0
  Reset : Inport  Port=3  OutDataType=sfix(16)  OutScaling=2^0
  Constant : Constant  Value=0  OutDataTypeMode=single  OutDataType=fixdt(1, 16)  OutScaling=2^0  OutDataTypeStr=single
  Convert to acceleration : Gain  Gain=1/mass  ParameterDataType=sfix(16)  ParameterScaling=2^0  OutDataType=sfix(16)  OutScaling=2^0
  Discrete-Time Integrator1 : DiscreteIntegrator  ExternalReset=level  SampleTime=-1  OutDataType=fixdt(1, 16)  OutScaling=2^0  ICPrevOutput=DiscIntNeverNeededParam  ICPrevScaledInput=DiscIntNeverNeededParam
  Product1 : Product  OutDataType=sfix(16)  OutScaling=2^0  RndMeth=Zero
  Product3 : Product  OutDataType=sfix(16)  OutScaling=2^0  RndMeth=Zero
  Trigonometric Function1 : Trigonometry  OutputSignalType=real
  Trigonometric Function2 : Trigonometry  Operator=cos  OutputSignalType=real
  myMux1 : Stateflow chart  TreatAsAtomicUnit=on
  Velocity : Outport  OutDataType=sfix(16)  OutScaling=2^0
  wires:
  Reset/1 -> Discrete-Time Integrator1/2
  Convert to acceleration/1 -> Discrete-Time Integrator1/1
  Discrete-Time Integrator1/1 -> Product3/1, Product1/1
  heading/1 -> Trigonometric Function2/1, Trigonometric Function1/1
  Trigonometric Function2/1 -> Product3/2
  myMux1/1(y) -> Velocity/1
  Product3/1 -> myMux1/1(u1)
  Product1/1 -> myMux1/2(u2)
  Trigonometric Function1/1 -> Product1/2
  Constant/1 -> myMux1/3(u3)
  X/1 -> Convert to acceleration/1

== system Boat_sim/Subsystem/Autonomous Controller/State Keeper & Estimator/GPS Estimator/Subsystem ==
  note: Multiply by .51444 to
      | convert knots to m/s
  gps : Inport
  Angle Conversion : uSimLib/Conversions/Angle Conversion  SystemSampleTime=-1  iu=deg  ou=rad
  Bus Selector : BusSelector  OutputSignals=sog
  Bus Selector1 : BusSelector  OutputSignals=cog
  Constant : Constant  Value=0  OutDataTypeMode=single  OutDataType=fixdt(1, 16)  OutScaling=2^0  OutDataTypeStr=single
  Gain : Gain  Gain=.5144444  ParameterDataType=fixdt(1, 16)  ParameterScaling=2^0  OutDataType=fixdt(1, 16)  OutScaling=2^0
  Mux : Mux  Inputs=3
  Product : Product  OutDataTypeMode=single  OutDataType=fixdt(1, 16)  OutScaling=2^0  OutDataTypeStr=single  RndMeth=Zero
  Product1 : Product  OutDataTypeMode=single  OutDataType=fixdt(1, 16)  OutScaling=2^0  OutDataTypeStr=single  RndMeth=Zero
  Reorder : Subsystem
  Trigonometric Function : Trigonometry
  Trigonometric Function1 : Trigonometry  Operator=cos
  velocity : Outport
  heading : Outport  Port=2
  pos : Outport  Port=3
  time : Outport  Port=4
  wires:
  Gain/1 -> Product1/1, Product/1
  gps/1 -> Reorder/1(In1), Bus Selector/1, Bus Selector1/1
  Bus Selector1/1 -> Angle Conversion/1  "<cog>"
  Trigonometric Function/1 -> Product/2
  Trigonometric Function1/1 -> Product1/2
  Product1/1 -> Mux/1
  Product/1 -> Mux/2
  Constant/1 -> Mux/3
  Mux/1 -> velocity/1
  Angle Conversion/1 -> heading/1, Trigonometric Function/1, Trigonometric Function1/1
  Bus Selector/1 -> Gain/1  "<sog>"
  Reorder/1(pos) -> pos/1
  Reorder/2(time) -> time/1

== system Boat_sim/Subsystem/Autonomous Controller/Throttle Command/Mux Everything/Build speed command ==
  CC : Inport  OutDataType=sfix(16)  OutScaling=2^0
  Constant : Constant  OutDataTypeMode=uint8  OutDataType=sfix(16)  OutScaling=2^0  OutDataTypeStr=uint8
  Constant1 : Constant  Value=0  OutDataTypeMode=uint8  OutDataType=sfix(16)  OutScaling=2^0  OutDataTypeStr=uint8
  Constant2 : Constant  Value=0  OutDataTypeMode=uint8  OutDataType=sfix(16)  OutScaling=2^0  OutDataTypeStr=uint8
  Constant3 : Constant  Value=5  OutDataTypeMode=uint8  OutDataType=sfix(16)  OutScaling=2^0  OutDataTypeStr=uint8
  Mux : Mux  Inputs=5
  uint16 to uchar : Subsystem  AncestorBlock=uSimLib/Conversions/uint16 to uchar
  msg : Outport  OutDataType=sfix(16)  OutScaling=2^0
  wires:
  uint16 to uchar/1(uchar) -> Mux/3
  Constant/1 -> Mux/1
  Constant3/1 -> Mux/2
  Mux/1 -> msg/1
  Constant1/1 -> Mux/4
  Constant2/1 -> Mux/5
  CC/1 -> uint16 to uchar/1(ushort)

== system Boat_sim/Subsystem/Autonomous Controller/State Keeper & Estimator/GPS Estimator/Subsystem/Reorder ==
  In1 : Inport
  Angle Conversion : uSimLib/Conversions/Angle Conversion  SystemSampleTime=-1  iu=deg  ou=rad
  Angle Conversion1 : uSimLib/Conversions/Angle Conversion  SystemSampleTime=-1  iu=deg  ou=rad
  Bias : Bias  Bias=2000
  Bus Selector : BusSelector  OutputSignals=latitude,longitude,year,month,day,hour,minute,second
  Constant : Constant  Value=0  OutDataTypeMode=single  OutDataType=fixdt(1, 16)  OutScaling=2^0  OutDataTypeStr=single
  Data Type Conversion{1..8} (8 alike) : DataTypeConversion  OutDataTypeMode=single  OutDataType=fixdt(1, 16)  OutScaling=2^0  OutDataTypeStr=single
  Mux : Mux  Inputs=7
  Mux1 : Mux  Inputs=3
  Phase shift2 : Constant  Value=-8  OutDataTypeMode=single  OutDataType=sfix(16)  OutScaling=2^0  OutDataTypeStr=single
  Scope : Scope
  pos : Outport
  time : Outport  Port=2
  wires:
  Bus Selector/1 -> Data Type Conversion8/1  "<latitude>"
  Bus Selector/2 -> Data Type Conversion7/1  "<longitude>"
  Data Type Conversion1/1 -> Bias/1
  Bias/1 -> Mux/1
  Data Type Conversion2/1 -> Mux/2
  Bus Selector/3 -> Data Type Conversion1/1  "<year>"
  Bus Selector/4 -> Data Type Conversion2/1  "<month>"
  Bus Selector/5 -> Data Type Conversion3/1  "<day>"
  Bus Selector/6 -> Data Type Conversion4/1  "<hour>"
  Bus Selector/7 -> Data Type Conversion5/1  "<minute>"
  Bus Selector/8 -> Data Type Conversion6/1  "<second>"
  Data Type Conversion3/1 -> Mux/3
  Data Type Conversion4/1 -> Mux/4
  Data Type Conversion5/1 -> Mux/5
  Data Type Conversion6/1 -> Mux/6
  Phase shift2/1 -> Mux/7
  In1/1 -> Bus Selector/1
  Mux/1 -> time/1
  Angle Conversion/1 -> Scope/1, Mux1/1
  Angle Conversion1/1 -> Mux1/2
  Constant/1 -> Mux1/3
  Mux1/1 -> pos/1
  Data Type Conversion7/1 -> Angle Conversion1/1
  Data Type Conversion8/1 -> Angle Conversion/1

== system Boat_sim/Subsystem/Autonomous Controller/Throttle Command/Mux Everything/Build speed command/uint16 to uchar ==
  ushort : Inport
  Data Type Conversion : DataTypeConversion  OutDataTypeMode=uint16  OutDataType=fixdt(1, 16)  OutScaling=2^0  OutDataTypeStr=uint16  ConvertRealWorld=Stored Integer (SI)  RndMeth=Simplest
  Extract Bits1 : simulink/Logic and Bit Operations/Extract Bits  SystemSampleTime=-1  bitsToExtract=Upper half  numBits=8  bitIdxRange=[0 7]  outScalingMode=Treat bit field as an integer
  Extract Bits2 : simulink/Logic and Bit Operations/Extract Bits  SystemSampleTime=-1  bitsToExtract=Lower half  numBits=8  bitIdxRange=[0 7]  outScalingMode=Treat bit field as an integer
  Mux : Mux  Inputs=2
  uchar : Outport  OutDataType=fixdt(1, 16)  OutScaling=2^0
  wires:
  Mux/1 -> uchar/1
  Extract Bits2/1 -> Mux/2
  Extract Bits1/1 -> Mux/1
  ushort/1 -> Data Type Conversion/1
  Data Type Conversion/1 -> Extract Bits1/1, Extract Bits2/1

== matlab function HIL Interface/Build HIL sentence/Pack ==
  data: a input double; y output double; b input double; c input double; d input double; e input double; f input double
function y = fcn(a, b, c, d, e, f)
%#eml

y = zeros(46, 1, 'uint8');
y(1) = a;
y(2) = b;
y(3:43) = c;
y(44) = d;
y(45) = e;
y(46) = f;

== matlab function Plant/Get GPS/Embedded MATLAB Function1 ==
  data: cog output double; Vn input double; Ve input double
function cog = getCOG(Vn, Ve)
% This block supports an embeddable subset of the MATLAB language.
% See the help menu for details. 

cog = atan2(Ve,Vn);
if cog < 0;
    cog = cog + 2*pi;
end

== matlab function Subsystem/Autonomous Controller/State Keeper & Estimator/GPS Estimator/Calculate local position via velocity integral between true GPS updates ==
  data: latLonAlt input single size=[3 1]; localPosition output single; newData input boolean size=1; reset input boolean size=1; resetIntegrator output boolean size=1
function [localPosition,resetIntegrator] = estimateGPS(latLonAlt, newData, reset)
%#eml
% INPUTS:
% latLonAlt - the latitude, longitude, and altitude of the vehicle from GPS
% newData - A boolean signal specifying whether latLonAlt holds new data
% reset - A global reset boolean trigger.

% OUTPUTS:
% localPosition is the local position of the vehicle in relation to a recorded
% starting location in North-East-Down coordinates.
% resetIntegrator will reset the velocity integrator that's calculating the
% local position in between GPS reads.

persistent startingPosition lastKnownPosition newDataCounter;

% Reset everything on first startup or when a global reset is triggered
if isempty(startingPosition) || reset
    startingPosition = zeros(3, 1, 'single');
end
if isempty(lastKnownPosition) || reset
    lastKnownPosition = zeros(3, 1, 'single');
end
if isempty(newDataCounter) || reset
    newDataCounter = zeros(1, 1, 'uint8');
end

% Reset the integrator if a global reset is called
if reset
    resetIntegrator = true;
else
    resetIntegrator = false;
end

% Wait for 5 valid GPS inputs before latching a starting point
if newDataCounter < 5
    % Check that we have valid data before latching it.
    if newData && latLonAlt(1) ~= 0 && latLonAlt(2) ~= 0
        newDataCounter = newDataCounter + 1;
        startingPosition = latLonAlt;
    end
    
    % We output all 0s while we're waiting
    localPosition = zeros(3, 1, 'single');
else
    % Latch a new position if one's been received. Also reset the integrator
    % for this timestep as we have a "truth" position now.
    if newData
        lastKnownPosition = latLonAlt;
        resetIntegrator = true;
    end
    
    % Calculate the difference between the starting position and the last
    % known position.
    localPosition = dg2lg(startingPosition, latLonAlt);
end

% Not certain how this works or where I got it from.
function out = dg2lg(u1, u2)

dlat = (u2(1) - u1(1))*pi/180;
dlon = (u2(2) - u1(2))*pi/180;
lat = u1(1)*pi/180;
h = u2(3);
a = 6378137;
e2 = 0.00669437999014;

v=a./sqrt(1-e2.*sin(lat).^2);
r=v.*(1-e2)./(1-e2.*sin(lat).^2);
dx=dlat.*(r+h);
dy=dlon.*cos(lat).*(v+h);

% Map into North-East-Down coordinates
out = [dy;-dx;0];

== matlab function Subsystem/Autonomous Controller/State Keeper & Estimator/GPS Estimator/Outputs/myMux1 ==
  data: u1 input double; y output double; u2 input double; u3 input double
function y = myMux(u1, u2, u3)
y = [u1(1); u2(1); u3(1)];
